simulink model "open_loop_3d"  (Simulink 7.9)
settings: Solver=FixedStepDiscrete  StartTime=0.0  StopTime=tend  FixedStep=params.th  MaxStep=0.01  RelTol=1e-6  AbsTol=1e-3
values from neighbouring files (symbols this model uses):
  delta_cp = 0    [ctrl_design.m]    (also in ctrl_design_v2.m)
  delta_k = 12    [ctrl_design.m]    (also in ctrl_design_v2.m)
  delta_pot = 50    [ctrl_design.m]    (also in ctrl_design_v2.m = 0)
  delta_vel = 0    [ctrl_design.m]    (also in ctrl_design_v2.m = 5e-05)
  t_step = 0    [ctrl_design.m]    (also in ctrl_design_v2.m)
undefined symbols (not defined in the file or in its folder): params
settings Model: Creator=puri  LastModifiedBy=Manu
settings CodeAppCC: CustomSymbolStrType=$N$R$M_T
settings GRTTargetCC: CodeReplacementLibrary=None  CPPClassGenCompliant=on

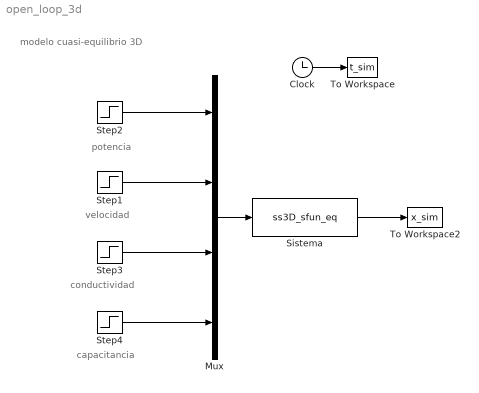
== system open_loop_3d ==
  note: modelo cuasi-equilibrio 3D
  note: potencia
  note: velocidad
  note: conductividad
  note: capacitancia
  Clock : Clock
  Mux : Mux
  Sistema : S-Function  FunctionName=ss3D_sfun_eq  EnableBusSupport=off
      settings: DeleteFcn=shh = get(0,'ShowHiddenHandles');set(0,'ShowHiddenHandles','on');if ~isempty(findobj('type','figure','name','dblcart1 Animation'));close('dblcart1 Animation'); end;set(0,'ShowHiddenHandles',shh);
  Step1 : Step  Time=t_step  Before=params.v_nom  After=params.v_nom + delta_vel  SampleTime=0
  Step2 : Step  Time=t_step  Before=params.Pot_nom  After=params.Pot_nom + delta_pot  SampleTime=0
  Step3 : Step  Time=t_step  Before=params.ks  After=params.ks + delta_k  SampleTime=0
  Step4 : Step  Time=t_step  Before=params.cs  After=params.cs + delta_cp  SampleTime=0
  To Workspace : ToWorkspace  VariableName=t_sim  SampleTime=-1
  To Workspace2 : ToWorkspace  VariableName=x_sim  SampleTime=-1
  wires:
  Mux/1 -> Sistema/1
  Sistema/1 -> To Workspace2/1
  Clock/1 -> To Workspace/1
  Step2/1 -> Mux/1
  Step1/1 -> Mux/2
  Step3/1 -> Mux/3
  Step4/1 -> Mux/4
